simulink model "robot011"  (R2016a)
settings: Solver=FixedStepDiscrete  StartTime=0.0  StopTime=inf  FixedStep=0.001  RelTol=1e-3
libraries: SIA_Robot_Toolbox x13
settings Model: SimulationMode=external  Creator=Administrator  LastModifiedBy=qinsi
settings OptimizationCC: OptimizeModelRefInitCode=on  LifeSpan=Inf
settings RTWCC: SystemTargetFile=linux_ert_target.tlc  GenCodeOnly=on  MakeCommand=make_rtw CC=gcc  TemplateMakefile=linux_ert_target.tmf  Description=Linux Embedded Real-Time target  RetainRTWFile=on
settings CodeAppCC: ForceParamTrailComments=on  IgnoreCustomStorageClasses=off  OperatorAnnotations=on  SimulinkDataObjDesc=on  SFDataObjDesc=on  MATLABFcnDesc=on  InsertBlockDesc=on  MATLABSourceComments=on
settings STFCustomTargetCC: CombineOutputUpdateFcns=on  ERTCustomFileBanners=on  SupportNonInlinedSFcns=off  MATLABClassNameForMDSCustomization=Simulink.SoftwareTarget.ERTCustomization  GRTInterface=off  SystemTargetFile=linux_ert_target.tlc
settings ERTTargetCC: ParMdlRefBuildCompliant=off  CompOptLevelCompliant=off  ConcurrentExecutionCompliant=off  ERTFirstTimeCompliant=off  SupportContinuousTime=on  ModelStepFunctionPrototypeControlCompliant=off  CPPClassGenCompliant=off  UseToolchainInfoCompliant=off  ExtMode=on  ExtModeMexArgs='192.168.0.99' 1 17725  ERTSrcFileBannerTemplate=linux_ert_target_code_template.cgt  ERTHdrFileBannerTemplate=linux_ert_target_code_template.cgt  ERTDataSrcFileTemplate=linux_ert_target_code_template.cgt  ERTDataHdrFileTemplate=linux_ert_target_code_template.cgt  ERTCustomFileTemplate=linux_ert_target_generate_main.tlc

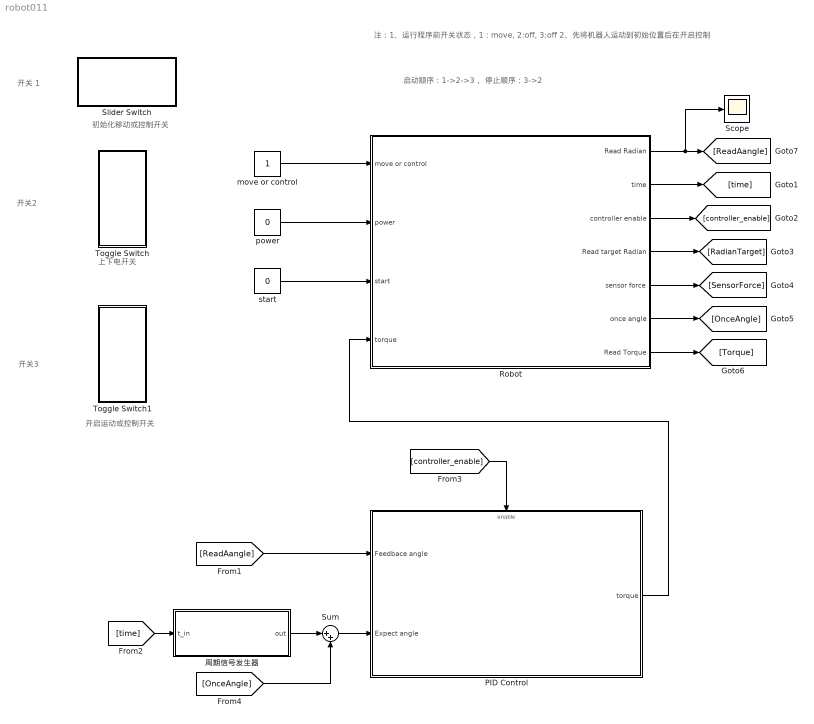
== system robot011 ==
  note: 启动顺序：1->2->3，
      | 停止顺序：3->2
  note: 开关 1
  note: 注：1、运行程序前开关状态，1：move, 2:off, 3:off
      | 2、先将机器人运动到初始位置后在开启控制
  note: 开启运动或控制开关
  note: 上下电开关
  note: 初始化移动或控制开关
  note: 开关2
  note: 开关3
  PID Control : Subsystem
  Robot : Subsystem  mask(模块说明){move_joint=[0 0 0 0 0 0]}
      mask prompts: move_joint "move_joint(rad)"
      mask help: 不需要更改该模块内部程序。
  Scope : Scope
  Slider Switch : Subsystem  DialogController=hmiCreateDDGDialog  IsWebBlock=on  mask(MWDashboardBlock){webBlockId=0f822388-ba08-46af-9411-5149fe75d7e0, webBlockType=sliderswitch, ShowInLibBrowser=on, ShowInitialText=on, HMISrcModelName=robot002A}
      mask prompts: webBlockId "WebBlock Id"; webBlockType "WebBlock Type"; HMISrcModelName "Source Model"
      mask Help: helpview([docroot '/mapfiles/simulink.map'], 'hmi_slider_switch')
      mask Display:
      | if strcmp(get_param(bdroot(gcb),'BlockDiagramType'), 'library')
      |     image([(matlabroot) '/toolbox/simulink/hmi/icons/SliderSwitch.png']);
      | end
  Sum : Sum  Inputs=|++
  Toggle Switch : Subsystem  DialogController=hmiCreateDDGDialog  IsWebBlock=on  mask(MWDashboardBlock){webBlockId=d5829285-805e-4e9c-a75a-8a5066d51c6d, webBlockType=toggleswitch, ShowInLibBrowser=on, ShowInitialText=on, HMISrcModelName=robot002A}
      mask prompts: webBlockId "WebBlock Id"; webBlockType "WebBlock Type"; HMISrcModelName "Source Model"
      mask Help: helpview([docroot '/mapfiles/simulink.map'], 'hmi_toggle_switch')
      mask Display:
      | if strcmp(get_param(bdroot(gcb),'BlockDiagramType'), 'library')
      |     image([(matlabroot) '/toolbox/simulink/hmi/icons/ToggleSwitch.png']);
      | end
  Toggle Switch1 : Subsystem  DialogController=hmiCreateDDGDialog  IsWebBlock=on  mask(MWDashboardBlock){webBlockId=c25893f3-06ef-48df-8be0-be34984d502e, webBlockType=toggleswitch, ShowInLibBrowser=on, ShowInitialText=on, HMISrcModelName=robot002A}
      mask prompts: webBlockId "WebBlock Id"; webBlockType "WebBlock Type"; HMISrcModelName "Source Model"
      mask Help: helpview([docroot '/mapfiles/simulink.map'], 'hmi_toggle_switch')
      mask Display:
      | if strcmp(get_param(bdroot(gcb),'BlockDiagramType'), 'library')
      |     image([(matlabroot) '/toolbox/simulink/hmi/icons/ToggleSwitch.png']);
      | end
  move or control : Constant
  power : Constant  Value=0
  start : Constant  Value=0
  周期信号发生器 : MATLAB Function  TreatAsAtomicUnit=on  mask{Amplitude=[0 0 0 0 0 1], Bias=[0 0 0 0 0 0], Frequency=[0.1 0.1 0.1 0.1 0.1 0.1], Phase=[0 0 0 0 0 0]}
  wires:
  move or control/1 -> Robot/1(move or control)
  power/1 -> Robot/2(power)
  Robot/2(time) -> [time]
  Robot/3(controller enable) -> [controller_enable]
  Robot/4(Read target Radian) -> [RadianTarget]
  Robot/5(sensor force) -> [SensorForce]
  Robot/6(once angle) -> [OnceAngle]
  Robot/7(Read Torque) -> [Torque]
  [controller_enable] -> PID Control/Enable
  start/1 -> Robot/3(start)
  Robot/1(Read Radian) -> Scope/1, [ReadAangle]
  PID Control/1(torque) -> Robot/4(torque)
  [time] -> 周期信号发生器/1(t_in)
  周期信号发生器/1(out) -> Sum/1
  [ReadAangle] -> PID Control/1(Feedbace angle)
  Sum/1 -> PID Control/2(Expect angle)
  [OnceAngle] -> Sum/2

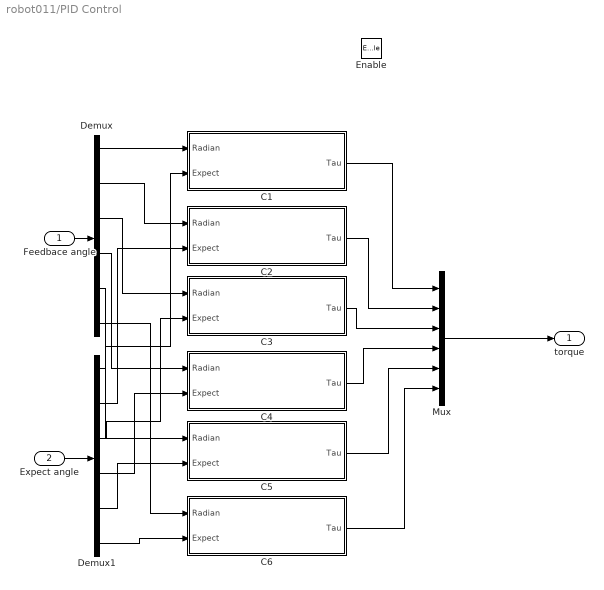
== system robot011/PID Control ==
  Feedbace angle : Inport
  Expect angle : Inport  Port=2
  Enable : EnablePort
  C1 : Subsystem
  C2 : Subsystem
  C3 : Subsystem
  C4 : Subsystem
  C5 : Subsystem
  C6 : Subsystem
  Demux : Demux  Outputs=6
  Demux1 : Demux  Outputs=6
  Mux : Mux  Inputs=6
  torque : Outport
  wires:
  C1/1(Tau) -> Mux/1
  Demux1/6 -> C6/2(Expect)
  Demux1/5 -> C5/2(Expect)
  Feedbace angle/1 -> Demux/1
  Demux/6 -> C6/1(Radian)
  C6/1(Tau) -> Mux/6
  Demux1/3 -> C3/2(Expect)
  Demux/2 -> C2/1(Radian)
  Demux/5 -> C5/1(Radian)
  C4/1(Tau) -> Mux/4
  Demux1/2 -> C2/2(Expect)
  Demux/1 -> C1/1(Radian)
  Demux/3 -> C3/1(Radian)
  Mux/1 -> torque/1
  C5/1(Tau) -> Mux/5
  Demux1/4 -> C4/2(Expect)
  C2/1(Tau) -> Mux/2
  Demux/4 -> C4/1(Radian)
  C3/1(Tau) -> Mux/3
  Demux1/1 -> C1/2(Expect)
  Expect angle/1 -> Demux1/1

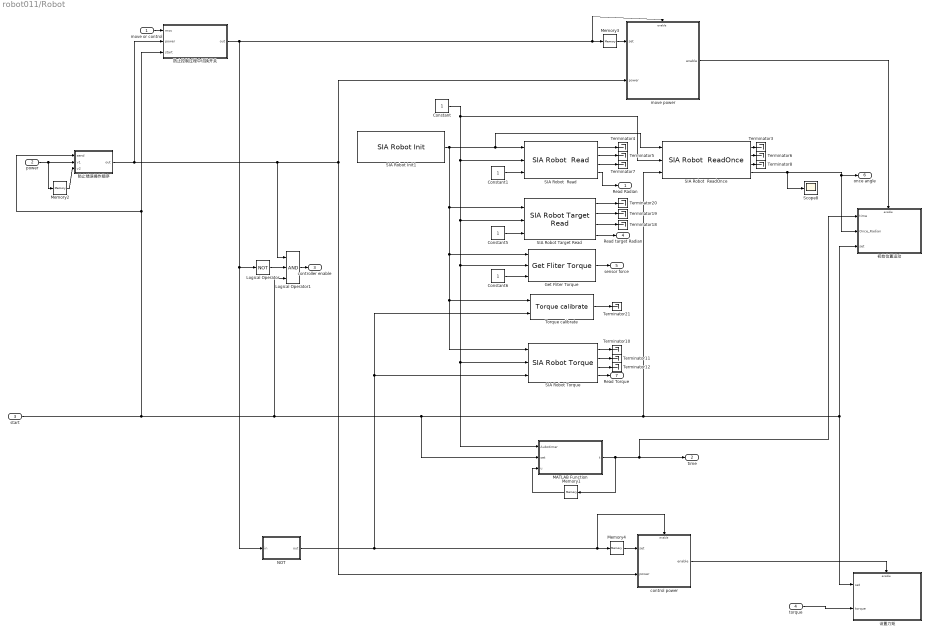
== system robot011/Robot ==
  move or control : Inport
  power : Inport  Port=2
  start : Inport  Port=3
  torque : Inport  Port=4
  " Torque calibrate" : SIA_Robot_Toolbox/Sensor/ Torque calibrate
  Constant{,1,5..6} (4 alike) : Constant
  Get Fliter Torque : SIA_Robot_Toolbox/Sensor/Get Fliter Torque  p_buf_num_sensor=20
  Logical Operator : Logic  Operator=NOT  AllPortsSameDT=off  OutDataTypeStr=boolean
  Logical Operator1 : Logic  Inputs=3  AllPortsSameDT=off  OutDataTypeStr=boolean
  MATLAB Function : MATLAB Function  TreatAsAtomicUnit=on
  Memory{1..4} (4 alike) : Memory
  NOT : MATLAB Function  TreatAsAtomicUnit=on
  SIA Robot  Read : SIA_Robot_Toolbox/Robot Interface/SIA Robot  Read  g_Axisnum=6
  SIA Robot  ReadOnce : SIA_Robot_Toolbox/Robot Interface/SIA Robot  ReadOnce  g_Axisnum=6
  SIA Robot Init1 : SIA_Robot_Toolbox/Robot System Tool/SIA Robot Init  p_grip_init=on  p_pop=COBOTGRAB  p_para=/dev/ttyUSB0  p_egm_init=on  p_robot_index=0  p_guide_type=0  p_input_type=1  p_cycle_times=2
  SIA Robot Target Read : SIA_Robot_Toolbox/Robot Interface/SIA Robot Target Read
  SIA Robot Torque : SIA_Robot_Toolbox/Robot Interface/SIA Robot Torque  Parameter1=6
  Scope8 : Scope
  Terminator{3..8,10..12,18..21} (13 alike) : Terminator
  control power : Subsystem
  move power : Subsystem
  初始位置运动 : Subsystem
  设置力矩 : Subsystem
  防止控制过程中切换开关 : MATLAB Function  TreatAsAtomicUnit=on
  防止错误操作顺序 : MATLAB Function  TreatAsAtomicUnit=on
  Read Radian : Outport
  time : Outport  Port=2
  controller enable : Outport  Port=3
  Read target Radian : Outport  Port=4
  sensor force : Outport  Port=5
  once angle : Outport  Port=6
  Read Torque : Outport  Port=7
  wires:
  Constant/1 -> SIA Robot  ReadOnce/2, SIA Robot  Read/2, SIA Robot Target Read/2, SIA Robot Torque/2, MATLAB Function/1(Aubotimer), Get Fliter Torque/2
  SIA Robot Init1/1 -> Get Fliter Torque/1, SIA Robot Torque/1, " Torque calibrate"/1, SIA Robot Target Read/1, SIA Robot  ReadOnce/1, SIA Robot  Read/1
  Constant1/1 -> SIA Robot  Read/3
  Memory1/1 -> MATLAB Function/3(u)
  SIA Robot  ReadOnce/1 -> Terminator3/1
  SIA Robot  Read/4 -> Read Radian/1
  SIA Robot  ReadOnce/4 -> Scope8/1, 初始位置运动/2(Once_Radian), once angle/1
  MATLAB Function/1(t) -> 初始位置运动/1(time), time/1, Memory1/1
  SIA Robot  Read/1 -> Terminator4/1
  SIA Robot  Read/2 -> Terminator5/1
  SIA Robot  ReadOnce/2 -> Terminator6/1
  SIA Robot  Read/3 -> Terminator7/1
  SIA Robot  ReadOnce/3 -> Terminator8/1
  防止错误操作顺序/1(out) -> 防止控制过程中切换开关/2(power), Logical Operator1/1, control power/2(power), move power/2(power)
  防止控制过程中切换开关/1(out) -> NOT/1(in), Logical Operator/1, move power/Enable, Memory3/1
  NOT/1(out) -> SIA Robot Torque/3, " Torque calibrate"/2, Memory4/1, control power/Enable
  move or control/1 -> 防止控制过程中切换开关/1(moc)
  Memory2/1 -> 防止错误操作顺序/3(v2)
  power/1 -> Memory2/1, 防止错误操作顺序/2(v1)
  Logical Operator1/1 -> controller enable/1
  Logical Operator/1 -> Logical Operator1/2
  Constant5/1 -> SIA Robot Target Read/3
  SIA Robot Target Read/4 -> Read target Radian/1
  SIA Robot Target Read/3 -> Terminator18/1
  SIA Robot Target Read/2 -> Terminator19/1
  SIA Robot Target Read/1 -> Terminator20/1
  Constant6/1 -> Get Fliter Torque/3
  Get Fliter Torque/1 -> sensor force/1
  " Torque calibrate"/1 -> Terminator21/1
  move power/1(enable) -> 初始位置运动/Enable
  control power/1(enable) -> 设置力矩/Enable
  start/1 -> 防止控制过程中切换开关/3(start), 防止错误操作顺序/1(send), Logical Operator1/3, MATLAB Function/2(set), 设置力矩/1(set), 初始位置运动/3(set), SIA Robot  ReadOnce/3
  SIA Robot Torque/3 -> Terminator12/1
  SIA Robot Torque/2 -> Terminator11/1
  SIA Robot Torque/1 -> Terminator10/1
  SIA Robot Torque/4 -> Read Torque/1
  torque/1 -> 设置力矩/2(torque)
  Memory3/1 -> move power/1(set)
  Memory4/1 -> control power/1(set)

== system robot011/Slider Switch ==

== system robot011/Toggle Switch ==

== system robot011/Toggle Switch1 ==

== system robot011/PID Control/C1 ==
  Radian : Inport
  Expect : Inport  Port=2
  Tau : Outport

== system robot011/PID Control/C2 ==
  Radian : Inport
  Expect : Inport  Port=2
  Tau : Outport

== system robot011/PID Control/C3 ==
  Radian : Inport
  Expect : Inport  Port=2
  Tau : Outport

== system robot011/PID Control/C4 ==
  Radian : Inport
  Expect : Inport  Port=2
  Tau : Outport

== system robot011/PID Control/C5 ==
  Radian : Inport
  Expect : Inport  Port=2
  Tau : Outport

== system robot011/PID Control/C6 ==
  Radian : Inport
  Expect : Inport  Port=2
  Tau : Outport

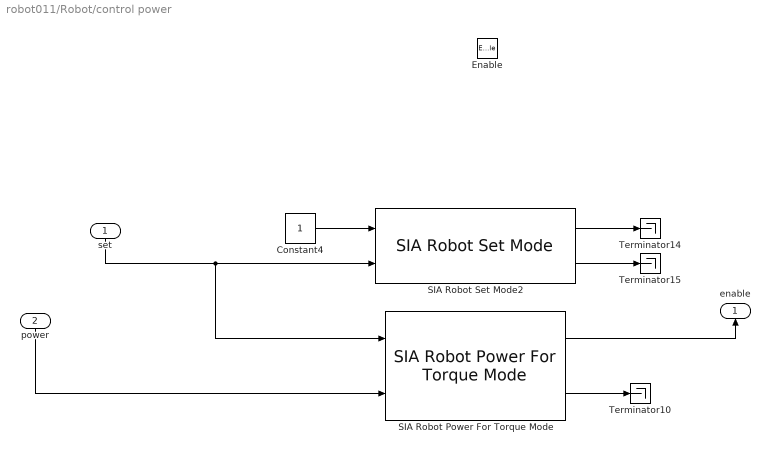
== system robot011/Robot/control power ==
  set : Inport
  power : Inport  Port=2
  Enable : EnablePort
  Constant4 : Constant
  SIA Robot Power For Torque Mode : SIA_Robot_Toolbox/Robot System Tool/SIA Robot Power For Torque Mode  Axis_1=off  Axis_2=off  Axis_3=off  Axis_4=off  Axis_5=off  Axis_6=on
      link override S-Function Builder: Parameters=Axis_1,Axis_2,Axis_3,Axis_4,Axis_5,Axis_6
  SIA Robot Set Mode2 : SIA_Robot_Toolbox/Robot Interface/SIA Robot Set Mode  Axis_1=off  Axis_2=off  Axis_3=off  Axis_4=off  Axis_5=off  Axis_6=on
      link override S-Function Builder: Parameters=Axis_1,Axis_2,Axis_3,Axis_4,Axis_5,Axis_6
  Terminator10 : Terminator
  Terminator14 : Terminator
  Terminator15 : Terminator
  enable : Outport
  wires:
  SIA Robot Power For Torque Mode/1 -> enable/1
  SIA Robot Set Mode2/2 -> Terminator15/1
  SIA Robot Set Mode2/1 -> Terminator14/1
  SIA Robot Power For Torque Mode/2 -> Terminator10/1
  Constant4/1 -> SIA Robot Set Mode2/1
  set/1 -> SIA Robot Set Mode2/2, SIA Robot Power For Torque Mode/1
  power/1 -> SIA Robot Power For Torque Mode/2

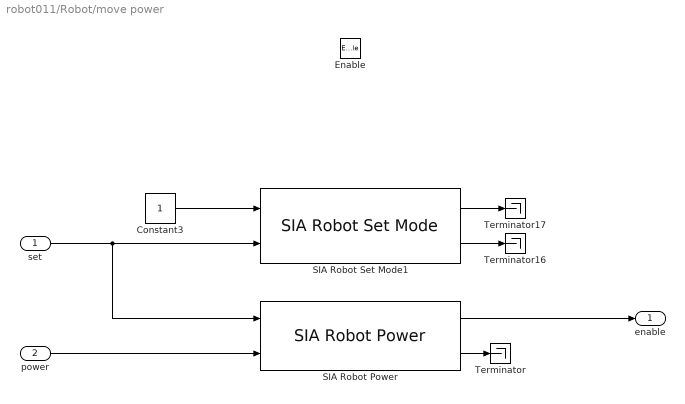
== system robot011/Robot/move power ==
  set : Inport
  power : Inport  Port=2
  Enable : EnablePort
  Constant3 : Constant
  SIA Robot Power : SIA_Robot_Toolbox/Robot System Tool/SIA Robot Power  r0=on  r1=off
  SIA Robot Set Mode1 : SIA_Robot_Toolbox/Robot Interface/SIA Robot Set Mode  m_mode=速度模式  Axis_all=off  Axis_1=off  Axis_2=off  Axis_3=off  Axis_4=off  Axis_5=off  Axis_6=off
      link override S-Function Builder: Parameters=Axis_1,Axis_2,Axis_3,Axis_4,Axis_5,Axis_6
  Terminator : Terminator
  Terminator16 : Terminator
  Terminator17 : Terminator
  enable : Outport
  wires:
  power/1 -> SIA Robot Power/2
  SIA Robot Power/2 -> Terminator/1
  Constant3/1 -> SIA Robot Set Mode1/1
  SIA Robot Power/1 -> enable/1
  SIA Robot Set Mode1/2 -> Terminator16/1
  SIA Robot Set Mode1/1 -> Terminator17/1
  set/1 -> SIA Robot Power/1, SIA Robot Set Mode1/2

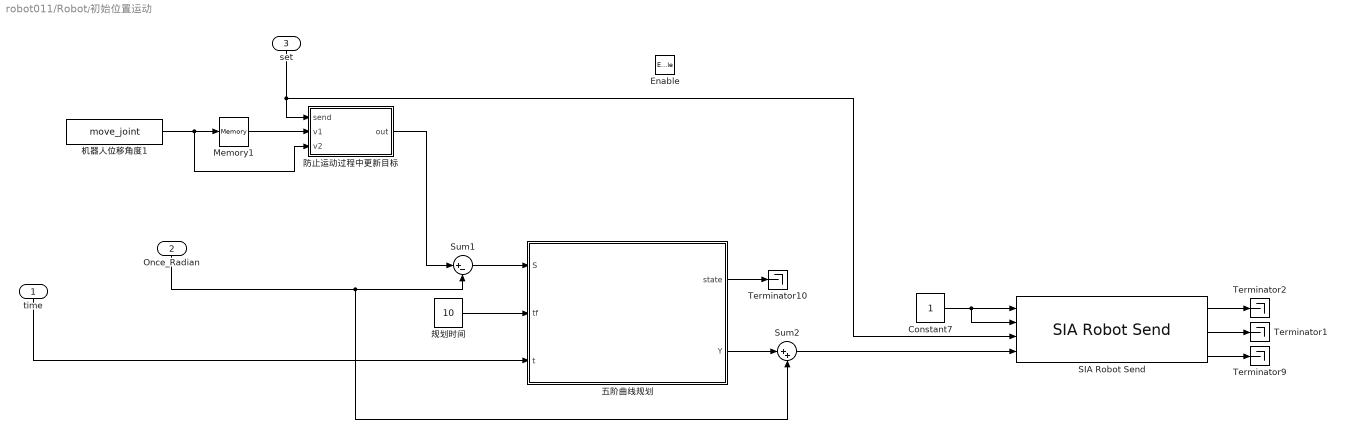
== system robot011/Robot/初始位置运动 ==
  time : Inport
  Once_Radian : Inport  Port=2
  set : Inport  Port=3
  Enable : EnablePort
  Constant7 : Constant
  Memory1 : Memory  X0=[0 0 0 0 0 0]
  SIA Robot Send : SIA_Robot_Toolbox/Robot Interface/SIA Robot Send  g_Axisnum=6
  Sum1 : Sum  Inputs=|+-
  Sum2 : Sum  Inputs=|++
  Terminator{1..2,9..10} (4 alike) : Terminator
  五阶曲线规划 : Subsystem
  机器人位移角度1 : Constant  Value=move_joint
  规划时间 : Constant  Value=10
  防止运动过程中更新目标 : MATLAB Function  TreatAsAtomicUnit=on
  wires:
  五阶曲线规划/2(Y) -> Sum2/1
  Once_Radian/1 -> Sum2/2, Sum1/2
  规划时间/1 -> 五阶曲线规划/2(tf)
  Sum1/1 -> 五阶曲线规划/1(S)
  五阶曲线规划/1(state) -> Terminator10/1
  time/1 -> 五阶曲线规划/3(t)
  Sum2/1 -> SIA Robot Send/4
  set/1 -> SIA Robot Send/3, 防止运动过程中更新目标/1(send)
  防止运动过程中更新目标/1(out) -> Sum1/1
  机器人位移角度1/1 -> 防止运动过程中更新目标/3(v2), Memory1/1
  Memory1/1 -> 防止运动过程中更新目标/2(v1)
  Constant7/1 -> SIA Robot Send/2, SIA Robot Send/1
  SIA Robot Send/3 -> Terminator9/1
  SIA Robot Send/2 -> Terminator1/1
  SIA Robot Send/1 -> Terminator2/1

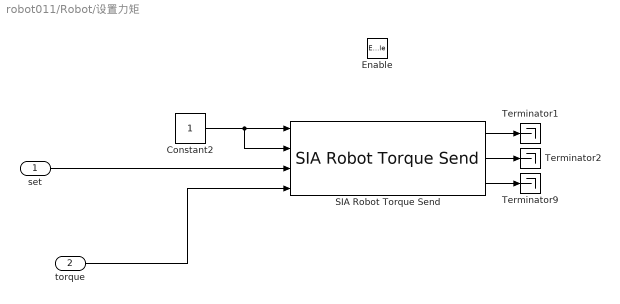
== system robot011/Robot/设置力矩 ==
  set : Inport
  torque : Inport  Port=2
  Enable : EnablePort
  Constant2 : Constant
  SIA Robot Torque Send : SIA_Robot_Toolbox/Robot Interface/SIA Robot Torque Send
  Terminator1 : Terminator
  Terminator2 : Terminator
  Terminator9 : Terminator
  wires:
  Constant2/1 -> SIA Robot Torque Send/2, SIA Robot Torque Send/1
  torque/1 -> SIA Robot Torque Send/4
  SIA Robot Torque Send/3 -> Terminator9/1
  SIA Robot Torque Send/1 -> Terminator1/1
  set/1 -> SIA Robot Torque Send/3
  SIA Robot Torque Send/2 -> Terminator2/1

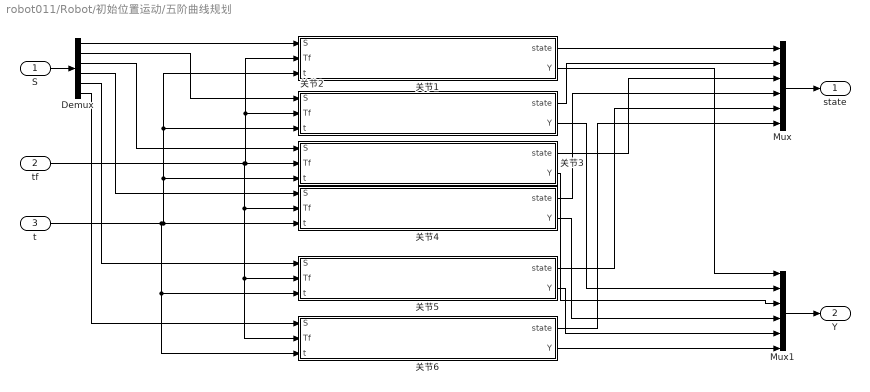
== system robot011/Robot/初始位置运动/五阶曲线规划 ==
  S : Inport
  tf : Inport  Port=2
  t : Inport  Port=3
  Demux : Demux  Outputs=6
  Mux : Mux  Inputs=6
  Mux1 : Mux  Inputs=6
  关节1 : Subsystem
  关节2 : Subsystem
  关节3 : Subsystem
  关节4 : Subsystem
  关节5 : Subsystem
  关节6 : Subsystem
  state : Outport
  Y : Outport  Port=2
  wires:
  关节6/1(state) -> Mux/6
  关节5/1(state) -> Mux/5
  Mux/1 -> state/1
  关节6/2(Y) -> Mux1/6
  关节5/2(Y) -> Mux1/5
  关节4/2(Y) -> Mux1/4
  关节3/2(Y) -> Mux1/3
  关节2/2(Y) -> Mux1/2
  Mux1/1 -> Y/1
  Demux/1 -> 关节1/1(S)
  S/1 -> Demux/1
  关节4/1(state) -> Mux/4
  关节2/1(state) -> Mux/2
  关节3/1(state) -> Mux/3
  关节1/1(state) -> Mux/1
  关节1/2(Y) -> Mux1/1
  Demux/2 -> 关节2/1(S)
  Demux/3 -> 关节3/1(S)
  Demux/4 -> 关节4/1(S)
  Demux/5 -> 关节5/1(S)
  Demux/6 -> 关节6/1(S)
  tf/1 -> 关节6/2(Tf), 关节5/2(Tf), 关节4/2(Tf), 关节3/2(Tf), 关节1/2(Tf), 关节2/2(Tf)
  t/1 -> 关节6/3(t), 关节5/3(t), 关节4/3(t), 关节3/3(t), 关节1/3(t), 关节2/3(t)

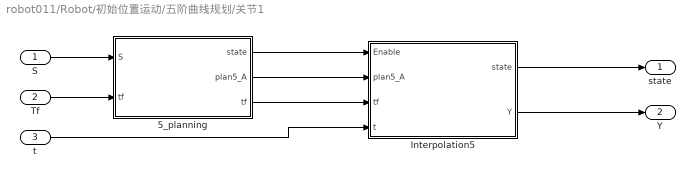
== system robot011/Robot/初始位置运动/五阶曲线规划/关节1 ==
  S : Inport
  Tf : Inport  Port=2
  t : Inport  Port=3
  5_planning : MATLAB Function  TreatAsAtomicUnit=on  mask{g_vs=0, g_ve=0, g_as=0, g_ae=0}
      mask prompts: g_vs "初始速度"; g_ve "末速度"; g_as "初始加速度"; g_ae "末加速度"
  Interpolation5 : MATLAB Function  TreatAsAtomicUnit=on
  state : Outport
  Y : Outport  Port=2
  wires:
  Interpolation5/1(state) -> state/1
  Interpolation5/2(Y) -> Y/1
  Tf/1 -> 5_planning/2("tf ")
  5_planning/3(tf) -> Interpolation5/3(tf)
  5_planning/2(plan5_A) -> Interpolation5/2(plan5_A)
  5_planning/1(state) -> Interpolation5/1(Enable)
  S/1 -> 5_planning/1(S)
  t/1 -> Interpolation5/4(t)

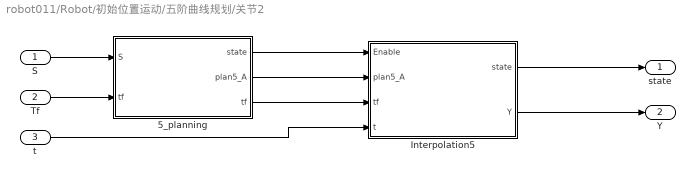
== system robot011/Robot/初始位置运动/五阶曲线规划/关节2 ==
  S : Inport
  Tf : Inport  Port=2
  t : Inport  Port=3
  5_planning : MATLAB Function  TreatAsAtomicUnit=on  mask{g_vs=0, g_ve=0, g_as=0, g_ae=0}
      mask prompts: g_vs "初始速度"; g_ve "末速度"; g_as "初始加速度"; g_ae "末加速度"
  Interpolation5 : MATLAB Function  TreatAsAtomicUnit=on
  state : Outport
  Y : Outport  Port=2
  wires:
  t/1 -> Interpolation5/4(t)
  S/1 -> 5_planning/1(S)
  5_planning/1(state) -> Interpolation5/1(Enable)
  5_planning/2(plan5_A) -> Interpolation5/2(plan5_A)
  5_planning/3(tf) -> Interpolation5/3(tf)
  Tf/1 -> 5_planning/2("tf ")
  Interpolation5/2(Y) -> Y/1
  Interpolation5/1(state) -> state/1

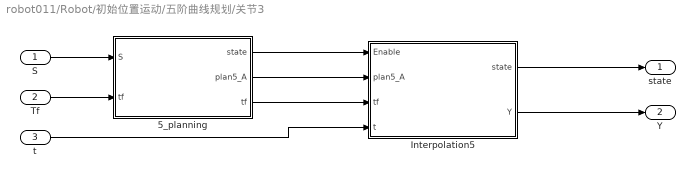
== system robot011/Robot/初始位置运动/五阶曲线规划/关节3 ==
  S : Inport
  Tf : Inport  Port=2
  t : Inport  Port=3
  5_planning : MATLAB Function  TreatAsAtomicUnit=on  mask{g_vs=0, g_ve=0, g_as=0, g_ae=0}
      mask prompts: g_vs "初始速度"; g_ve "末速度"; g_as "初始加速度"; g_ae "末加速度"
  Interpolation5 : MATLAB Function  TreatAsAtomicUnit=on
  state : Outport
  Y : Outport  Port=2
  wires:
  Interpolation5/1(state) -> state/1
  Interpolation5/2(Y) -> Y/1
  Tf/1 -> 5_planning/2("tf ")
  5_planning/3(tf) -> Interpolation5/3(tf)
  5_planning/2(plan5_A) -> Interpolation5/2(plan5_A)
  5_planning/1(state) -> Interpolation5/1(Enable)
  S/1 -> 5_planning/1(S)
  t/1 -> Interpolation5/4(t)

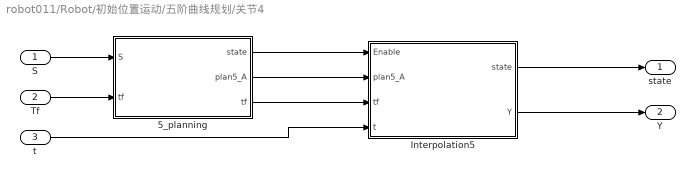
== system robot011/Robot/初始位置运动/五阶曲线规划/关节4 ==
  S : Inport
  Tf : Inport  Port=2
  t : Inport  Port=3
  5_planning : MATLAB Function  TreatAsAtomicUnit=on  mask{g_vs=0, g_ve=0, g_as=0, g_ae=0}
      mask prompts: g_vs "初始速度"; g_ve "末速度"; g_as "初始加速度"; g_ae "末加速度"
  Interpolation5 : MATLAB Function  TreatAsAtomicUnit=on
  state : Outport
  Y : Outport  Port=2
  wires:
  t/1 -> Interpolation5/4(t)
  S/1 -> 5_planning/1(S)
  5_planning/1(state) -> Interpolation5/1(Enable)
  5_planning/2(plan5_A) -> Interpolation5/2(plan5_A)
  5_planning/3(tf) -> Interpolation5/3(tf)
  Tf/1 -> 5_planning/2("tf ")
  Interpolation5/2(Y) -> Y/1
  Interpolation5/1(state) -> state/1

== system robot011/Robot/初始位置运动/五阶曲线规划/关节5 ==
  S : Inport
  Tf : Inport  Port=2
  t : Inport  Port=3
  5_planning : MATLAB Function  TreatAsAtomicUnit=on  mask{g_vs=0, g_ve=0, g_as=0, g_ae=0}
      mask prompts: g_vs "初始速度"; g_ve "末速度"; g_as "初始加速度"; g_ae "末加速度"
  Interpolation5 : MATLAB Function  TreatAsAtomicUnit=on
  state : Outport
  Y : Outport  Port=2
  wires:
  Interpolation5/1(state) -> state/1
  Interpolation5/2(Y) -> Y/1
  Tf/1 -> 5_planning/2("tf ")
  5_planning/3(tf) -> Interpolation5/3(tf)
  5_planning/2(plan5_A) -> Interpolation5/2(plan5_A)
  5_planning/1(state) -> Interpolation5/1(Enable)
  S/1 -> 5_planning/1(S)
  t/1 -> Interpolation5/4(t)

== system robot011/Robot/初始位置运动/五阶曲线规划/关节6 ==
  S : Inport
  Tf : Inport  Port=2
  t : Inport  Port=3
  5_planning : MATLAB Function  TreatAsAtomicUnit=on  mask{g_vs=0, g_ve=0, g_as=0, g_ae=0}
      mask prompts: g_vs "初始速度"; g_ve "末速度"; g_as "初始加速度"; g_ae "末加速度"
  Interpolation5 : MATLAB Function  TreatAsAtomicUnit=on
  state : Outport
  Y : Outport  Port=2
  wires:
  t/1 -> Interpolation5/4(t)
  S/1 -> 5_planning/1(S)
  5_planning/1(state) -> Interpolation5/1(Enable)
  5_planning/2(plan5_A) -> Interpolation5/2(plan5_A)
  5_planning/3(tf) -> Interpolation5/3(tf)
  Tf/1 -> 5_planning/2("tf ")
  Interpolation5/2(Y) -> Y/1
  Interpolation5/1(state) -> state/1

== matlab function robot011/Robot/MATLAB Function ==
  data: Aubotimer input; set input; u input; t output
  function t = Aubotime(Aubotimer,set,u)
%#codegen
persistent flag;
if isempty(flag)
flag = 0;
end
if(set == 1)   
    t = u+0.001;
else
    t = 0;
end

== matlab function robot011/Robot/初始位置运动/五阶曲线规划/关节2/5_planning ==
  data: S input; tf input; state output; plan5_A output; g_vs parameter; g_ve parameter; tf output; g_as parameter; g_ae parameter
function [state, plan5_A,tf] =planning5( S,tf,g_vs, g_ve, g_as, g_ae)
% 五次多项式算法主程序
% vs初始速度m/min,ve末速度m/min
% as初始加速度，ae末加速度
% S总位移m,tf为规划时间
% 基础插补规划函数
% 五次多项式速度规划
    a=zeros(1,6);
    a(1) = 0 ;
    a(2) = g_vs ;
    a(3) = g_as/2;
    a(4) = (20*S - (8*g_ve + 12 * g_vs )*tf - (3*g_as - g_ae)*tf^2)/(2*tf^3);
    a(5) = (-30*S + (14*g_ve + 16 * g_vs )*tf + (3*g_as - 2*g_ae)*tf^2)/(2*tf^4);
    a(6) = (12*S - 6*(g_ve + g_vs )*tf + (g_ae - g_as)*tf^2)/(2*tf^5);
    
    state1 = 1;
    state = state1;
    plan5_A = a;
    tf =tf ;
end

== matlab function robot011/Robot/初始位置运动/五阶曲线规划/关节1/5_planning ==
  data: S input; tf input; state output; plan5_A output; g_vs parameter; g_ve parameter; tf output; g_as parameter; g_ae parameter
function [state, plan5_A,tf] =planning5( S,tf,g_vs, g_ve, g_as, g_ae)
% 五次多项式算法主程序
% vs初始速度m/min,ve末速度m/min
% as初始加速度，ae末加速度
% S总位移m,tf为规划时间
% 基础插补规划函数
% 五次多项式速度规划
    a=zeros(1,6);
    a(1) = 0 ;
    a(2) = g_vs ;
    a(3) = g_as/2;
    a(4) = (20*S - (8*g_ve + 12 * g_vs )*tf - (3*g_as - g_ae)*tf^2)/(2*tf^3);
    a(5) = (-30*S + (14*g_ve + 16 * g_vs )*tf + (3*g_as - 2*g_ae)*tf^2)/(2*tf^4);
    a(6) = (12*S - 6*(g_ve + g_vs )*tf + (g_ae - g_as)*tf^2)/(2*tf^5);
    
    state1 = 1;
    state = state1;
    plan5_A = a;
    tf =tf ;
end

== matlab function robot011/Robot/初始位置运动/五阶曲线规划/关节2/Interpolation5 ==
  data: state output; Enable input; Y output; plan5_A input; tf input; t input
function [state, Y]  = Interpolate5(Enable,plan5_A,tf,t)
%% input
a0 = plan5_A(1);
a1 = plan5_A(2);
a2 = plan5_A(3);
a3 = plan5_A(4);
a4 = plan5_A(5);
a5 = plan5_A(6);
Y = 0;
%% output
if Enable == 1
    if t <=tf
    Y = a0 + a1*t + a2*t^2 + a3*t^3 + a4*t^4 + a5*t^5; 
    state =1;
    else
    Y = a0 + a1*tf + a2*tf^2 + a3*tf^3 + a4*tf^4 + a5*tf^5;
    state = 1;
    end
else 
    Y = 0;
    state = 0;
end
end

== matlab function robot011/Robot/初始位置运动/五阶曲线规划/关节3/5_planning ==
  data: S input; tf input; state output; plan5_A output; g_vs parameter; g_ve parameter; tf output; g_as parameter; g_ae parameter
function [state, plan5_A,tf] =planning5( S,tf,g_vs, g_ve, g_as, g_ae)
% 五次多项式算法主程序
% vs初始速度m/min,ve末速度m/min
% as初始加速度，ae末加速度
% S总位移m,tf为规划时间
% 基础插补规划函数
% 五次多项式速度规划
    a=zeros(1,6);
    a(1) = 0 ;
    a(2) = g_vs ;
    a(3) = g_as/2;
    a(4) = (20*S - (8*g_ve + 12 * g_vs )*tf - (3*g_as - g_ae)*tf^2)/(2*tf^3);
    a(5) = (-30*S + (14*g_ve + 16 * g_vs )*tf + (3*g_as - 2*g_ae)*tf^2)/(2*tf^4);
    a(6) = (12*S - 6*(g_ve + g_vs )*tf + (g_ae - g_as)*tf^2)/(2*tf^5);
    
    state1 = 1;
    state = state1;
    plan5_A = a;
    tf =tf ;
end

== matlab function robot011/Robot/初始位置运动/五阶曲线规划/关节3/Interpolation5 ==
  data: state output; Enable input; Y output; plan5_A input; tf input; t input
function [state, Y]  = Interpolate5(Enable,plan5_A,tf,t)
%% input
a0 = plan5_A(1);
a1 = plan5_A(2);
a2 = plan5_A(3);
a3 = plan5_A(4);
a4 = plan5_A(5);
a5 = plan5_A(6);
Y = 0;
%% output
if Enable == 1
    if t <=tf
    Y = a0 + a1*t + a2*t^2 + a3*t^3 + a4*t^4 + a5*t^5; 
    state =1;
    else
    Y = a0 + a1*tf + a2*tf^2 + a3*tf^3 + a4*tf^4 + a5*tf^5;
    state = 1;
    end
else 
    Y = 0;
    state = 0;
end
end

== matlab function robot011/Robot/初始位置运动/五阶曲线规划/关节4/5_planning ==
  data: S input; tf input; state output; plan5_A output; g_vs parameter; g_ve parameter; tf output; g_as parameter; g_ae parameter
function [state, plan5_A,tf] =planning5( S,tf,g_vs, g_ve, g_as, g_ae)
% 五次多项式算法主程序
% vs初始速度m/min,ve末速度m/min
% as初始加速度，ae末加速度
% S总位移m,tf为规划时间
% 基础插补规划函数
% 五次多项式速度规划
    a=zeros(1,6);
    a(1) = 0 ;
    a(2) = g_vs ;
    a(3) = g_as/2;
    a(4) = (20*S - (8*g_ve + 12 * g_vs )*tf - (3*g_as - g_ae)*tf^2)/(2*tf^3);
    a(5) = (-30*S + (14*g_ve + 16 * g_vs )*tf + (3*g_as - 2*g_ae)*tf^2)/(2*tf^4);
    a(6) = (12*S - 6*(g_ve + g_vs )*tf + (g_ae - g_as)*tf^2)/(2*tf^5);
    
    state1 = 1;
    state = state1;
    plan5_A = a;
    tf =tf ;
end

== matlab function robot011/Robot/初始位置运动/五阶曲线规划/关节4/Interpolation5 ==
  data: state output; Enable input; Y output; plan5_A input; tf input; t input
function [state, Y]  = Interpolate5(Enable,plan5_A,tf,t)
%% input
a0 = plan5_A(1);
a1 = plan5_A(2);
a2 = plan5_A(3);
a3 = plan5_A(4);
a4 = plan5_A(5);
a5 = plan5_A(6);
Y = 0;
%% output
if Enable == 1
    if t <=tf
    Y = a0 + a1*t + a2*t^2 + a3*t^3 + a4*t^4 + a5*t^5; 
    state =1;
    else
    Y = a0 + a1*tf + a2*tf^2 + a3*tf^3 + a4*tf^4 + a5*tf^5;
    state = 1;
    end
else 
    Y = 0;
    state = 0;
end
end

== matlab function robot011/Robot/初始位置运动/五阶曲线规划/关节5/5_planning ==
  data: S input; tf input; state output; plan5_A output; g_vs parameter; g_ve parameter; tf output; g_as parameter; g_ae parameter
function [state, plan5_A,tf] =planning5( S,tf,g_vs, g_ve, g_as, g_ae)
% 五次多项式算法主程序
% vs初始速度m/min,ve末速度m/min
% as初始加速度，ae末加速度
% S总位移m,tf为规划时间
% 基础插补规划函数
% 五次多项式速度规划
    a=zeros(1,6);
    a(1) = 0 ;
    a(2) = g_vs ;
    a(3) = g_as/2;
    a(4) = (20*S - (8*g_ve + 12 * g_vs )*tf - (3*g_as - g_ae)*tf^2)/(2*tf^3);
    a(5) = (-30*S + (14*g_ve + 16 * g_vs )*tf + (3*g_as - 2*g_ae)*tf^2)/(2*tf^4);
    a(6) = (12*S - 6*(g_ve + g_vs )*tf + (g_ae - g_as)*tf^2)/(2*tf^5);
    
    state1 = 1;
    state = state1;
    plan5_A = a;
    tf =tf ;
end

== matlab function robot011/Robot/初始位置运动/五阶曲线规划/关节5/Interpolation5 ==
  data: state output; Enable input; Y output; plan5_A input; tf input; t input
function [state, Y]  = Interpolate5(Enable,plan5_A,tf,t)
%% input
a0 = plan5_A(1);
a1 = plan5_A(2);
a2 = plan5_A(3);
a3 = plan5_A(4);
a4 = plan5_A(5);
a5 = plan5_A(6);
Y = 0;
%% output
if Enable == 1
    if t <=tf
    Y = a0 + a1*t + a2*t^2 + a3*t^3 + a4*t^4 + a5*t^5; 
    state =1;
    else
    Y = a0 + a1*tf + a2*tf^2 + a3*tf^3 + a4*tf^4 + a5*tf^5;
    state = 1;
    end
else 
    Y = 0;
    state = 0;
end
end

== matlab function robot011/Robot/初始位置运动/五阶曲线规划/关节6/5_planning ==
  data: S input; tf input; state output; plan5_A output; g_vs parameter; g_ve parameter; tf output; g_as parameter; g_ae parameter
function [state, plan5_A,tf] =planning5( S,tf,g_vs, g_ve, g_as, g_ae)
% 五次多项式算法主程序
% vs初始速度m/min,ve末速度m/min
% as初始加速度，ae末加速度
% S总位移m,tf为规划时间
% 基础插补规划函数
% 五次多项式速度规划
    a=zeros(1,6);
    a(1) = 0 ;
    a(2) = g_vs ;
    a(3) = g_as/2;
    a(4) = (20*S - (8*g_ve + 12 * g_vs )*tf - (3*g_as - g_ae)*tf^2)/(2*tf^3);
    a(5) = (-30*S + (14*g_ve + 16 * g_vs )*tf + (3*g_as - 2*g_ae)*tf^2)/(2*tf^4);
    a(6) = (12*S - 6*(g_ve + g_vs )*tf + (g_ae - g_as)*tf^2)/(2*tf^5);
    
    state1 = 1;
    state = state1;
    plan5_A = a;
    tf =tf ;
end

== matlab function robot011/Robot/初始位置运动/五阶曲线规划/关节6/Interpolation5 ==
  data: state output; Enable input; Y output; plan5_A input; tf input; t input
function [state, Y]  = Interpolate5(Enable,plan5_A,tf,t)
%% input
a0 = plan5_A(1);
a1 = plan5_A(2);
a2 = plan5_A(3);
a3 = plan5_A(4);
a4 = plan5_A(5);
a5 = plan5_A(6);
Y = 0;
%% output
if Enable == 1
    if t <=tf
    Y = a0 + a1*t + a2*t^2 + a3*t^3 + a4*t^4 + a5*t^5; 
    state =1;
    else
    Y = a0 + a1*tf + a2*tf^2 + a3*tf^3 + a4*tf^4 + a5*tf^5;
    state = 1;
    end
else 
    Y = 0;
    state = 0;
end
end

== matlab function robot011/Robot/防止控制过程中切换开关 ==
  data: moc input; power input; start input; out output
  function out = move_control_deal(moc,power,start)
%#codegen
persistent flag;
if isempty(flag)
flag = 0;
end
persistent flag1;
if isempty(flag1)
flag1 = 0;
end

if ((0==power)&&(0==start))
   out=moc;
   flag1=moc;
else
    if (0==flag)
      flag1=moc;
    end
    out=flag1;
end

    flag=1;

  end

== matlab function robot011/Robot/初始位置运动/五阶曲线规划/关节1/Interpolation5 ==
  data: state output; Enable input; Y output; plan5_A input; tf input; t input
function [state, Y]  = Interpolate5(Enable,plan5_A,tf,t)
%% input
a0 = plan5_A(1);
a1 = plan5_A(2);
a2 = plan5_A(3);
a3 = plan5_A(4);
a4 = plan5_A(5);
a5 = plan5_A(6);
Y = 0;
%% output
if Enable == 1
    if t <=tf
    Y = a0 + a1*t + a2*t^2 + a3*t^3 + a4*t^4 + a5*t^5; 
    state =1;
    else
    Y = a0 + a1*tf + a2*tf^2 + a3*tf^3 + a4*tf^4 + a5*tf^5;
    state = 1;
    end
else 
    Y = 0;
    state = 0;
end
end

== matlab function robot011/Robot/防止错误操作顺序 ==
  data: send input; v1 input; out output; v2 input
function out  = update(send,v1,v2)
persistent flag;
if isempty(flag)
flag = 0;
end

persistent out_;
if isempty(out_)
out_ = 0;
end

if (0==v1)
    out=v1;
    flag=0;
else
    if ((v1>v2)&&(1==send))
       out=v2;
       out_=0;
       flag=1;
    else
        if (1==flag)
           out=0;
        else
           out=v1;
        end
    
    end
end
end

== matlab function robot011/周期信号发生器 ==
  data: Amplitude parameter; Bias parameter; Frequency parameter; Phase parameter; out output; t_in input
function out=PeriodicSignallGenerator(Amplitude,Bias,Frequency, Phase,t_in)

    [m,n]=size(Amplitude);
    Amplitude=reshape(Amplitude,m*n,1);
    Bias=reshape(Bias,m*n,1);
    Frequency=reshape(Frequency,m*n,1);
    Phase=reshape(Phase,m*n,1);
    %规划
	ss=zeros(m*n,1);
	se=Amplitude;
	vs=zeros(m*n,1);
	ve=zeros(m*n,1);
	as=zeros(m*n,1);
	ae=zeros(m*n,1);
	js=zeros(m*n,1);
	je=zeros(m*n,1);
	tend=0.25./Frequency;

	tf=tend;
	tf2=tend.*tend;
	tf3=tend.*tend.*tend;
	tf4=tend.*tend.*tend.*tend;
	tf5=tend.*tend.*tend.*tend.*tend;
	tf6=tend.*tend.*tend.*tend.*tend.*tend;
	tf7=tend.*tend.*tend.*tend.*tend.*tend.*tend;

	b1=se-js./6.0.*tf3 - as./2.0.*tf2 - vs.*tf - ss;
	b2=ve-js./2.0.*tf2 - as.*tf - vs;
	b3=ae-js.*tf - as;
	b4=je-js;

    a=zeros(m*n,8);
	a(:,1)=ss;
	a(:,2)=vs;
	a(:,3)=as./2.0;
	a(:,4)=js./6.0;
	a(:,5)=(35.*b1)./tf4 - (15.*b2)./tf3 + (5.*b3)./(2.*tf2) - b4./(6.*tf);
	a(:,6)=(39.*b2)./tf4 - (84.*b1)./tf5 - (7.*b3)./tf3 + b4./(2.*tf2);
	a(:,7)=(70.*b1)./tf6 - (34.*b2)./tf5 + (13.*b3)./(2.*tf4) - b4./(2.*tf3);
	a(:,8)=(10.*b2)./tf6 - (20.*b1)./tf7 - (2.*b3)./tf5 + b4./(6.*tf4);
    
    %
    t_=zeros(m*n,1);
    t=zeros(m*n,1);
    ts=1.0./Frequency;
	t14=ts./4.0;
	t24=ts./2.0;
	t34=3.*ts./4.0;
	t44=ts;
	
    sign_=ones(m*n,1);
    %   
    for k=1:m*n
        t(k)=t_in+Phase(k);
        if (t(k)<0)
            sign_(k)=-1;
            t(k)=-t(k);
        end
        t(k)=t(k)-floor(t(k)/ts(k))*ts(k);
        if ((t(k)>=0)&&(t(k)<t14(k)))
            t_(k)=t(k);
        end
        if ((t(k)>=t14(k))&&(t(k)<t24(k)))
             t_(k)=t24(k)-t(k); 
        end
        if((t(k)>=t24(k))&&(t(k)<t34(k)))
             t_(k)=t(k)-t24(k);
             sign_(k)=-1.*sign_(k);
        end
        if((t(k)>=t34(k)))
             t_(k)=t44(k)-t(k);
             sign_(k)=-1.*sign_(k);        
        end
    

        if (t(k)>tend(k))
            t(k)=tend(k);
        end
        if (t(k)<0)
            t(k)=0;
        end
    end

    
	t2=t_.*t_;
	t3=t_.*t_.*t_;
	t4=t_.*t_.*t_.*t_;
	t5=t_.*t_.*t_.*t_.*t_;
	t6=t_.*t_.*t_.*t_.*t_.*t_;
	t7=t_.*t_.*t_.*t_.*t_.*t_.*t_;

	out =a(:,8).*t7 + a(:,7).*t6 + a(:,6).*t5 + a(:,5).*t4 + a(:,4).*t3 + a(:,3).*t2 + a(:,2).*t + a(:,1);
	out=sign_.*out+Bias;

end

== matlab function robot011/Robot/NOT ==
  data: in input; out output
function out  = NOT(in)
if 0==in
    out=1;
else
    out=0;
end
  

end

== matlab function robot011/Robot/初始位置运动/防止运动过程中更新目标 ==
  data: send input; v1 input; out output; v2 input
function out  = update(send,v1,v2)
v1=reshape(v1,1,6);
v2=reshape(v2,1,6);
persistent flag;
if isempty(flag)
flag = 0;
end

persistent out_;
if isempty(out_)
out_ = zeros(1,6);
end

if (1==send)
    if ((norm(v1-v2)>0.001)||1==flag)
        out=out_;
        flag=1;
    else
        out=v2;
        out_=v2;
    end
else
    out=v2;
    out_=v2;
    flag=0;
end
end
